simulink model "SimScape_Simulation"  (R2019b)
settings: Solver=VariableStepAuto  StartTime=0.0  StopTime=37.0  RelTol=1e-3
model workspace: external: MAT-File C:\Users\Swoby\OneDrive\Plocha\DUM-E\V0.3\Overeni_Matlab\SimScape_Model\Robot_Arm_DataFile.mat (data not in the file)
undefined symbols (not defined in the file or in its folder): smiData, X, Y, Z
libraries: sm_lib x49, nesl_utility x12
(part 2 of 2)

== system SimScape_Simulation/Robot_Arm_Model/Wrist2/Wirst21_RIGID ==
  ReferenceFrame : sm_lib/Frames and Transforms/Reference Frame
  Solid : sm_lib/Body Elements/File Solid  ExtGeomFileName=Model\Wirst2_ipt.STEP  UnitType=FromFile  ExtGeomFileUnits=m  StepReaderType=HEX  ExportEntireGeometry=off  InertiaType=Custom  Mass=smiData.Solid(6).mass  MassUnits=kg  CenterOfMass=smiData.Solid(6).CoM  CenterOfMassUnits=mm  MomentsOfInertia=smiData.Solid(6).MoI  MomentsOfInertiaUnits=kg*mm^2  ProductsOfInertia=smiData.Solid(6).PoI  ProductsOfInertiaUnits=kg*mm^2  BasedOnType=DensityFromFile  Density=1000  DensityUnits=kg/m^3  DoExposeReferenceFrame=on  SerializedFrames=<Frames/>  GraphicType=FromGeometry  MarkerShape=Sphere  MarkerSize=10  GraphicVisPropType=SimpleVisualProperties  GraphicDiffuseColor=smiData.Solid(6).color  GraphicSpecularColor=[0.5 0.5 0.5 1.0]  GraphicAmbientColor=[0.15 0.15 0.15 1.0]  GraphicEmissiveColor=[0.0 0.0 0.0 1.0]  GraphicShininess=75  GraphicOpacity=smiData.Solid(6).opacity
  Transform : sm_lib/Frames and Transforms/Rigid Transform  TranslationMethod=Cartesian  TranslationStandardOffset=0  TranslationLengthUnit=mm  TranslationStandardAxis=+Z  TranslationCartesianOffset=smiData.RigidTransform(10).translation  TranslationROffset=0  TranslationROffsetUnits=m  TranslationZOffset=0  TranslationZOffsetUnits=m  TranslationThetaOffset=0  TranslationThetaOffsetUnits=deg  RotationMethod=ArbitraryAxis  RotationAngleUnits=rad  RotationStandardAxis=+Z  RotationAngle=smiData.RigidTransform(10).angle  RotationArbitraryAxis=smiData.RigidTransform(10).axis  FollAlignAxisA=+X  BaseAlignAxisA=+Y  FollAlignAxisB=+Y  BaseAlignAxisB=+Z  RotationSequenceAxes=FollowerAxes  RotationSequence=XYX  RotationSequenceAngles=[0 0 0]  RotationSequenceAnglesUnits=deg  RotationMatrix=[1 0 0; 0 1 0; 0 0 1]
  Transform1 : sm_lib/Frames and Transforms/Rigid Transform  TranslationMethod=Cartesian  TranslationStandardOffset=0  TranslationLengthUnit=mm  TranslationStandardAxis=+Z  TranslationCartesianOffset=smiData.RigidTransform(11).translation  TranslationROffset=0  TranslationROffsetUnits=m  TranslationZOffset=0  TranslationZOffsetUnits=m  TranslationThetaOffset=0  TranslationThetaOffsetUnits=deg  RotationMethod=ArbitraryAxis  RotationAngleUnits=rad  RotationStandardAxis=+Z  RotationAngle=smiData.RigidTransform(11).angle  RotationArbitraryAxis=smiData.RigidTransform(11).axis  FollAlignAxisA=+X  BaseAlignAxisA=+Y  FollAlignAxisB=+Y  BaseAlignAxisB=+Z  RotationSequenceAxes=FollowerAxes  RotationSequence=XYX  RotationSequenceAngles=[0 0 0]  RotationSequenceAnglesUnits=deg  RotationMatrix=[1 0 0; 0 1 0; 0 0 1]
  F : PMIOPort  Side=Left
  F1 : PMIOPort  Port=2  Side=Right
  connections:
  Solid/RConn1 -- ReferenceFrame/RConn1 -- Transform/LConn1 -- Transform1/LConn1
  Transform/RConn1 -- F/RConn1
  Transform1/RConn1 -- F1/RConn1

== matlab function SimScape_Simulation/MATLAB Function PKU ==
  data: R output size=[3 3]; t0 input; x output; t1 input; t2 input; t3 input; t4 input; t5 input; y output; z output
function [R,x,y,z]  = PKU(t0, t1, t2, t3, t4, t5)
% Parametrs
a0 = 0;
a1 = 0.265;
a2 = 0.22313448854;
a3 = 0.0995;
a4 = 0;
a5 = 0;

alpha0 = -pi/2;
alpha1 = 0;
alpha2 = 0;
alpha3 = -pi/2;
alpha4 = pi/2;
alpha5 = 0;

d0 = 0.1207;
d1 = 0;
d2 = 0;
d3 = 0;
d4 = 0.01355;
d5 = 0.200;

% initial value of thetas
th0 = 0;
th1 = 0;
th2 = deg2rad(211.6244444);
th3 = deg2rad(328.3756);
th4 = deg2rad(90);
th5 = 0;

% T01
T01 = TransformMatrix(d0, (t0+th0), a0, alpha0);
    
% T12
T12 = TransformMatrix(d1, (t1+th1), a1, alpha1);

% T23
T23 = TransformMatrix(d2, (t2+th2), a2, alpha2);

% T34
T34 = TransformMatrix(d3, (t3+th3), a3, alpha3);

% T45
T45 = TransformMatrix(d4, (t4+th4), a4, alpha4);

% T56  
T56 = TransformMatrix(d5, (t5+th5), a5, alpha5);

T06 = T01 * T12 * T23 * T34 * T45 * T56;

% neovereno

% T06
% r11 = sin(t0)*sin(t4)*cos(t5) - sin(t5)*sin(t1+t2+t3)*cos(t0) + cos(t0)*cos(t4)*cos(t5)*cos(t1+t2+t3);
% r21 = -sin(t0)*sin(t5)*sin(t1+t2+t3) + sin(t0)*cos(t4)*cos(t5)*cos(t1+t2+t3) - sin(t4)*cos(t0)*cos(t5);
% r31 = sin(t5)*cos(t1+t2+t3) - sin(t1+t2+t3)*cos(t4)*cos(t5);
% 
% r12 = -sin(t0)*sin(t4)*sin(t5) * sin(t5)*cos(t0)*cos(t4)*cos(t1+t2+t3) - sin(t1+t2+t3)*cos(t0)*cos(t5);
% r22 = -sin(t0)*sin(t5)*cos(t4)*cos(t1+t2+t3) - sin(t0)*sin(t1+t2+t3)*cos(t5) + sin(t4)*sin(t5)*cos(t0);
% r32 = sin(t5)*sin(t1+t2+t3)*cos(t4) - cos(t5)*cos(t1+t2+t3);
% 
% r13 = -sin(t0)*cos(t4) + sin(t4)*cos(t0)*cos(t1+t2+t3);
% r23 = sin(t0)*sin(t4)*cos(t1+t2+t3) + cos(t0)*cos(t4);
% r33 = -sin(t4)*sin(t1+t2+t3);
% 
% x = a1*cos(t0)*cos(t1) + a2*cos(t0)*cos(t1+t2) + a3*cos(t0)*cos(t1+t2+t3) - d4*sin(t1+t2+t3)*cos(t0) - d5*sin(t0)*cos(t4) + d5*sin(t4)*cos(t0)*cos(t1+t2+t3);
% y = a1*sin(t0)*cos(t1) + a2*sin(t0)*cos(t1+t2) + a3*sin(t0)*cos(t1+t2+t3) - d4*sin(t1+t2+t3)*sin(t0) + d5*cos(t0)*cos(t4) + d5*sin(t0)*sin(t4)*cos(t1+t2+t3);
% z = -a1*sin(t1) - a2*sin(t1+t2) - a3*sin(t1+t2+t3) + d0 - d4*cos(t1+t2+t3) - d5*sin(t4)*sin(t1+t2+t3);

R = T06(1:3, 1:3);
x = T06(1, 4);
y = T06(2, 4);
z = T06(3, 4);
end

== matlab function SimScape_Simulation/Robot_Arm_Model/MATLAB Function ==
  data: R input size=[3 3]; alpha output; beta output; gamma output
function [alpha,beta,gamma] = RotationMatrix2Angle(R)
% Function transform rotation matrix into euler angles
% R - rotation matrix 3x3 

[alpha,beta,gamma] = RotationMatrix2Angle(R);

end

== matlab function SimScape_Simulation/MATLAB Function2 ==
  data: R input; alpha output; beta output; gamma output
function [alpha,beta,gamma] = RotationMatrix2Angle(R)
% Function transform rotation matrix into euler angles
% R - rotation matrix 3x3 

[alpha,beta,gamma] = RotationMatrix2Angle(R);

end

== matlab function SimScape_Simulation/MATLAB Function IKU ==
  data: X input; t0 output; Y input; Z input; R input; t1 output; t2 output; t3 output; t4 output; t5 output
function [t0, t1, t2, t3, t4, t5]  = IKU(X, Y, Z, R)

%% Parametrs
% koeficient for D-H algoritm
a0 = 0;
a1 = 0.265;
a2 = 0.22313448854;
a3 = 0.0995;
a4 = 0;
a5 = 0;

alpha0 = -pi/2;
alpha1 = 0;
alpha2 = 0;
alpha3 = -pi/2;
alpha4 = pi/2;
alpha5 = 0;

d0 = 0.1207;
d1 = 0;
d2 = 0;
d3 = 0;
d4 = 0.01355;
d5 = 0.200;

%% IKU algoritm

O06 = [X; Y; Z];    % pozice koncoveho efektoru v 0. s.s.
O05 = O06 - d5 * R(1:3,3);  % pozice 5. s.s. v 0. s.s.

%% t0
t0 = atan2(-O05(2), -O05(1)); %% range +- pi

if(O05(1) > 0) % note-1
    t0 = pi+t0;
end
if(t0 > pi) % note-2
    t0 = t0-2*pi;
elseif(t0 < -pi)
    t0 = t0+2*pi;
end

%% compute (t1 + t2 + t3) t123
T05 = [[R,[X;Y;Z]];[0, 0, 0, 1]]; % transformation matrix from begin to end effector 
T01e = TransformMatrix(0, -t0, 0, 0); % only rotation about -t0 in Z axe 
T05e = T01e*T05; % <=> T15 = inv(T01)*T05; - estimate T05 for t0 = 0rad
t123 = -atan2(-T05e(3,3), -T05e(1,3)); % t1+t2+t3

%% compute t4
v = [-cos(t123); 0; sin(t123)]; % osa Z rotacni matice pro t4 = 0 rotovana podle osy y o t123
n = [sin(t123); 0; cos(t123)]; % normala k rovine po niz se muze rotovat kloub pro t4

% for t4 = pi/2 fail

t4 = -vecangle360(T05e(1:3,3), v, n);
%% compute t5
v = [-sin(-t123); 0; cos(-t123)]; % osa Y rotacni matice pro t4 = 0 rotovana podle osy y o t123
t5 = -vecangle360(T05e(1:3,2), v, T05e(1:3,3));


%% compute t1, t2, t3
O06e = T05e(1:3,4); % estimate [X,Y,Z] for t0 = 0 rad
O05e = O06e - d5 * T05e(1:3,3); % 5. s.s. pro t0 = 0 rad
O04e = O05e - d4 * v;

% t2
ct2 = ((-O04e(1)-a3*cos(t123))^2 + ((O04e(3)-d0) - a3*sin(t123))^2 - (a1^2+a2^2)) / (2*a1*a2); % cos(t2)
st2 = -sqrt(1-ct2^2); % sin(t2)

t2 = atan2(st2, ct2);

% t1
A = [-a2*sin(t2),   a2*cos(t2)+a1;
     a2*cos(t2)+a1,    a2*sin(t2)];
 
B = [-O04e(1)-a3*cos(t123);
     (O04e(3)-d0)-a3*sin(t123)]; 
 
g  = A\B; % = inv(A)*B

t1 = atan2(g(1),g(2))-pi;

% t3
t2 = t2 + 2.589652;
t3 = t123 - t1 - t2;

end

% note-1 
% bod O05 se ocitne za pocatkem ([0;0;0]) a mereni uhlu neplati

== matlab function SimScape_Simulation/Generator Uhlu motoru ==
  data: th0 output; t input; th1 output; th2 output; th3 output; th4 output; th5 output
function [th0, th1, th2, th3,th4, th5]  = Generator_Uhlu_Motoru(t)
    % t - time (seconds)
    % th - angles of motors
    
   % random parameters for generating movement
    q0 = 1; 
    q1 = 0.5;
    q2 = 0.3;
    q3 = 2;
    q4 = 3;
    q5 = 0.75;
    
    th0 = 0;
    th1 = 0;
    th2 = 0;
    th3 = 0;
    th4 = 0;
    th5 = 0;
    
%     if(t < 2*pi)
%         th0 = 0.5*pi*sin(t);
%     elseif(t > 2*pi && t < 4*pi)
%         th1 = 0.5*pi*sin(t);
%     elseif(t > 4*pi && t < 6*pi)
%         th2 = 0.5*pi*sin(t);
%     elseif(t > 6*pi && t < 8*pi)
%         th3 = 0.5*pi*sin(t);
%     elseif(t > 8*pi && t < 10*pi)
%         th4 = 0.5*pi*sin(t);
%     elseif(t > 10*pi && t < 12*pi)
%         th5 = 0.5*pi*sin(t);   
%     end

    th0 = 0.49*pi*sin(q0*t);
    th1 = 0.49*pi*cos(q1*t) - 0.49*pi;
    th2 = 0.40*pi*sin(q2*t);
    th3 = 0.49*pi*sin(q3*t);
    th4 = 0.40*pi*sin(q4*t); % on +- 0.5*pi is big problem for IKU
    th5 = 0.49*pi*sin(q5*t);

end
